simulink model "motor_pos_ctrl"  (R2023b)
settings: Solver=VariableStepAuto  StartTime=0.0  StopTime=1  RelTol=1e-3
InitFcn:
  | %%%%%%%%%%%%%%%%%%%%%%%%%%%%%%%%%%%%%%%%%%%%%%%%%
  | %motor parameters
  | %we dont know these yet
  | J = 1e-6; %intertia [kg * m^2]
  | Bm = 1e-6; %kinetic friction [N * m * s]
  | 
  | %from motor datasheet
  | Km = 0.011; %motor constant (back emf constant = torque constant)
  | Rw = 1.17; %motor electric resistance in ohms
  | Lw = 0.58E-3; %motor inductance in ohms
  | 
  | 
  | %admittance controller params
  | 
  | K = 1;
  | B = 1;
  | D = 1;
  | M = J;
  | M_inv = 1/J;
  | 
  | Kp =1
  | Ki = 1
  | Kd = 1
  | C = pid(Kp,Ki,Kd)
settings Model: Creator=you29  LastModifiedBy=you29

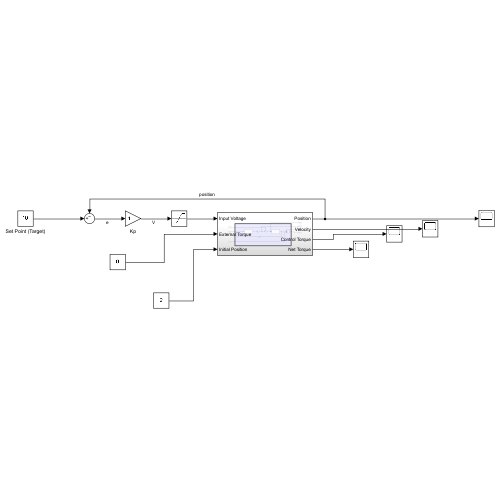
[thumbnail: Simulink's stored preview of the top-level diagram]
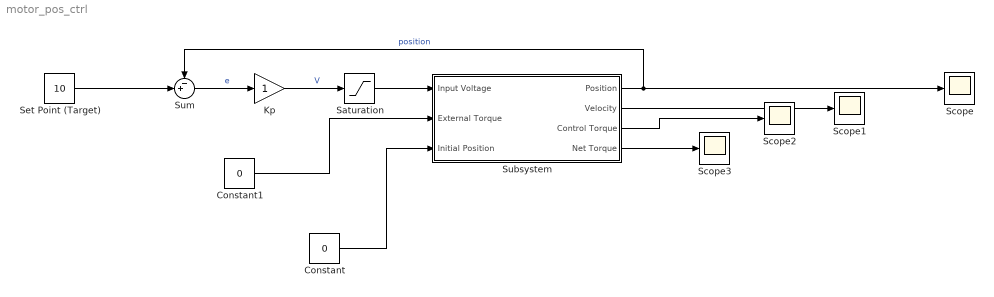
== system motor_pos_ctrl ==
  Constant : Constant  Value=0
  Constant1 : Constant  Value=0
  Kp : Gain
  Saturation : Saturate  UpperLimit=12  LowerLimit=-12
  Scope{,1..3} (4 alike) : Scope
  Set Point (Target) : Constant  Value=10
  Subsystem : Subsystem
  Sum : Sum  Inputs=-+|
  wires:
  Kp/1 -> Saturation/1  "V"
  Constant/1 -> Subsystem/3(Initial Position)
  Subsystem/1(Position) -> Scope/1, Sum/1  "position"
  Set Point (Target)/1 -> Sum/2
  Sum/1 -> Kp/1  "e"
  Constant1/1 -> Subsystem/2(External Torque)
  Subsystem/2(Velocity) -> Scope1/1
  Subsystem/3(Control Torque) -> Scope2/1
  Subsystem/4(Net Torque) -> Scope3/1
  Saturation/1 -> Subsystem/1(Input Voltage)

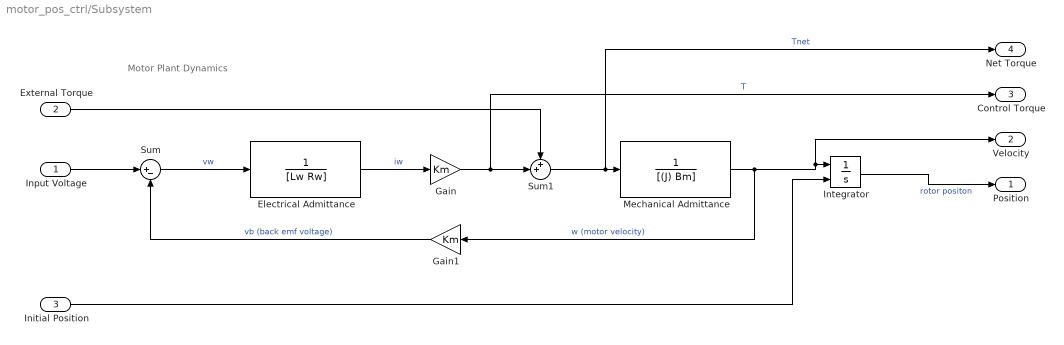
== system motor_pos_ctrl/Subsystem ==
  note: Motor Plant Dynamics
  Input Voltage : Inport
  External Torque : Inport  Port=2
  Initial Position : Inport  Port=3
  Electrical Admittance : TransferFcn  Denominator=[Lw Rw]
  Gain : Gain  Gain=Km
  Gain1 : Gain  Gain=Km
  Integrator : Integrator  InitialConditionSource=external
  Mechanical Admittance : TransferFcn  Denominator=[(J) Bm]
  Sum : Sum  Inputs=|+-
  Sum1 : Sum  Inputs=++|
  Position : Outport
  Velocity : Outport  Port=2
  Control Torque : Outport  Port=3
  Net Torque : Outport  Port=4
  wires:
  Input Voltage/1 -> Sum/1
  Mechanical Admittance/1 -> Velocity/1, Integrator/1, Gain1/1  "w (motor velocity)"
  Gain1/1 -> Sum/2  "vb (back emf voltage)"
  Integrator/1 -> Position/1  "rotor positon"
  Gain/1 -> Control Torque/1, Sum1/2  "T"
  Electrical Admittance/1 -> Gain/1  "iw"
  Sum/1 -> Electrical Admittance/1  "vw"
  Sum1/1 -> Net Torque/1, Mechanical Admittance/1  "Tnet"
  External Torque/1 -> Sum1/1
  Initial Position/1 -> Integrator/2
